simulink model "improved_hydroturbine"  (R2023b)
settings: Solver=VariableStepAuto  StartTime=0.0  StopTime=10.0  RelTol=1e-3
undefined symbols (not defined in the file or in its folder): ht
settings Model: Creator=tedbrekken  LastModifiedBy=tedbrekken

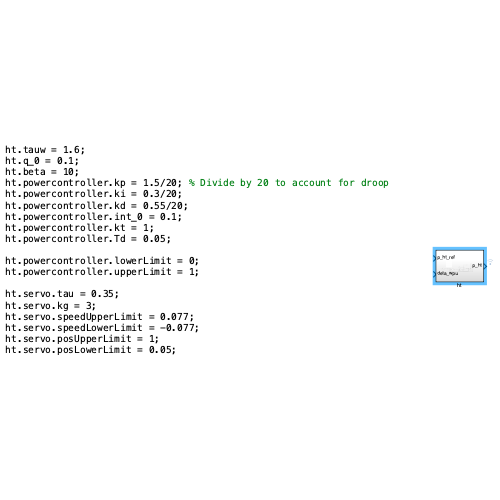
[thumbnail: Simulink's stored preview of the top-level diagram]
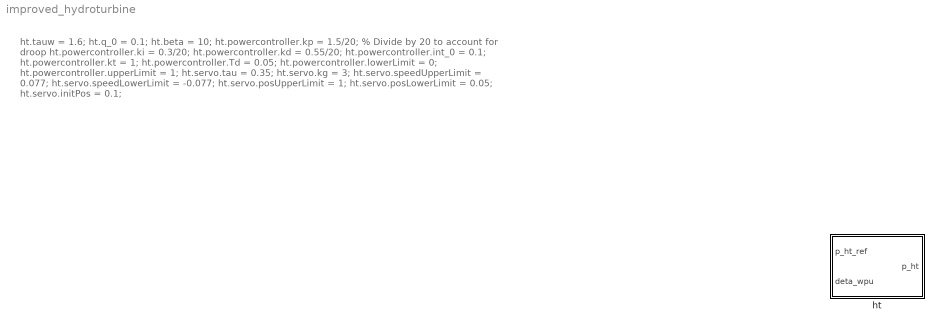
== system improved_hydroturbine ==
  note: ht.tauw = 1.6;
      | ht.q_0 = 0.1;
      | ht.beta = 10;
      | ht.powercontroller.kp = 1.5/20; % Divide by 20 to account for droop
      | ht.powercontroller.ki = 0.3/20;
      | ht.powercontroller.kd = 0.55/20;
      | ht.powercontroller.int_0 = 0.1;
      | ht.powercontroller.kt = 1;
      | ht.powercontroller.Td = 0.05;
      |
      | ht.powercontroller.lowerLimit = 0;
      | ht.powercontroller.upperLimit = 1;
      |
      | ht.servo.tau = 0.35;
      | ht.servo.kg = 3;
      | ht.servo.speedUpperLimit = 0.077;
      | ht.servo.speedLowerLimit = -0.077;
      | ht.servo.posUpperLimit = 1;
      | ht.servo.posLowerLimit = 0.05;
      | ht.servo.initPos = 0.1;
  ht : Subsystem

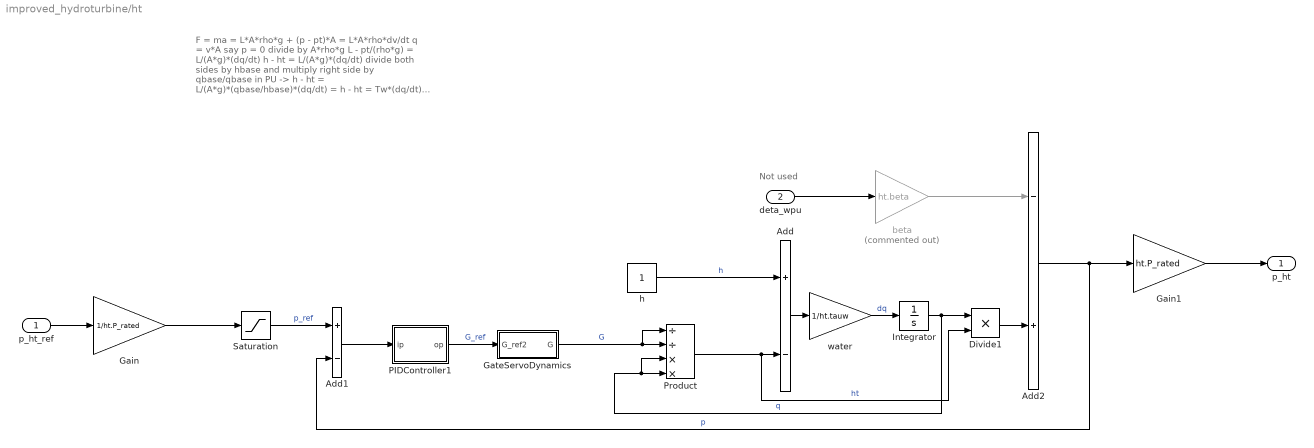
== system improved_hydroturbine/ht ==
  note: Not used
  note: F = ma = L*A*rho*g + (p - pt)*A = L*A*rho*dv/dt
      |
      | q = v*A
      |
      | say p = 0
      |
      | divide by A*rho*g
      |
      | L - pt/(rho*g) = L/(A*g)*(dq/dt)
      |
      | h - ht = L/(A*g)*(dq/dt)
      |
      | divide both sides by hbase and multiply right side by qbase/qbase
      |
      | in PU -> h - ht = L/(A*g)*(qbase/hbase)*(dq/dt) = h - ht = Tw*(dq/dt)
      |
      | ht = (q/G)^2
      |
      | pt = ht*q - beta*delta_w
      |
      | Increase in speed changes decreases relative angle of water attack on runner and decreases power
      | and vice versa
  p_ht_ref : Inport
  deta_wpu : Inport  Port=2
  Add : Sum  Inputs=+-
  Add1 : Sum  Inputs=+-
  Add2 : Sum  Inputs=-+
  Divide1 : Product  Inputs=**
  Gain : Gain  Gain=1/ht.P_rated
  Gain1 : Gain  Gain=ht.P_rated
  GateServoDynamics : Subsystem
  Integrator : Integrator  InitialCondition=ht.q_0
  PIDController1 : Subsystem  mask{kp=ht.powercontroller.kp, ki=ht.powercontroller.ki, kd=ht.powercontroller.kd, kt=ht.powercontroller.kt, Td=ht.powercontroller.Td, upperLimit=ht.powercontroller.upperLimit, lowerLimit=ht.powercontroller.lowerLimit, int_0=ht.powercontroller.int_0}
      mask prompts: kp "Proportional gain"; ki "Integral gain"; kd "Derivative gain"; kt "Windup gain"; Td "Derivative time constant"; upperLimit "Upper limit"; lowerLimit "Lower limit"; int_0 "Initial condition"
  Product : Product  Inputs=//**
  Saturation : Saturate  UpperLimit=1  LowerLimit=0
  beta : Gain  Commented=on  Gain=ht.beta
  h : Constant
  water : Gain  Gain=1/ht.tauw
  p_ht : Outport
  wires:
  water/1 -> Integrator/1  "dq"
  deta_wpu/1 -> beta/1
  beta/1 -> Add2/1
  Integrator/1 -> Product/3, Product/4, Divide1/1  "q"
  GateServoDynamics/1(G) -> Product/1, Product/2  "G"
  Product/1 -> Divide1/2, Add/2  "ht"
  Add/1 -> water/1
  h/1 -> Add/1  "h"
  Divide1/1 -> Add2/2
  PIDController1/1(op) -> GateServoDynamics/1(G_ref2)  "G_ref"
  Add2/1 -> Add1/2, Gain1/1  "p"
  Gain1/1 -> p_ht/1
  p_ht_ref/1 -> Gain/1
  Saturation/1 -> Add1/1  "p_ref"
  Gain/1 -> Saturation/1
  Add1/1 -> PIDController1/1(ip)

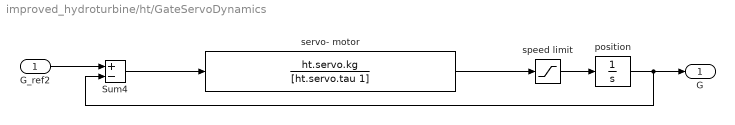
== system improved_hydroturbine/ht/GateServoDynamics ==
  G_ref2 : Inport
  Sum4 : Sum  Inputs=+-  InputSameDT=on  SaturateOnIntegerOverflow=on  OutDataTypeStr=Inherit: Same as first input
  position : Integrator  InitialCondition=ht.servo.initPos  LimitOutput=on  UpperSaturationLimit=ht.servo.posUpperLimit  LowerSaturationLimit=ht.servo.posLowerLimit
  servo- motor : TransferFcn  Numerator=ht.servo.kg  Denominator=[ht.servo.tau 1]
  speed limit : Saturate  UpperLimit=ht.servo.speedUpperLimit  LowerLimit=ht.servo.speedLowerLimit
  G : Outport
  wires:
  position/1 -> G/1, Sum4/2
  speed limit/1 -> position/1
  servo- motor/1 -> speed limit/1
  Sum4/1 -> servo- motor/1
  G_ref2/1 -> Sum4/1

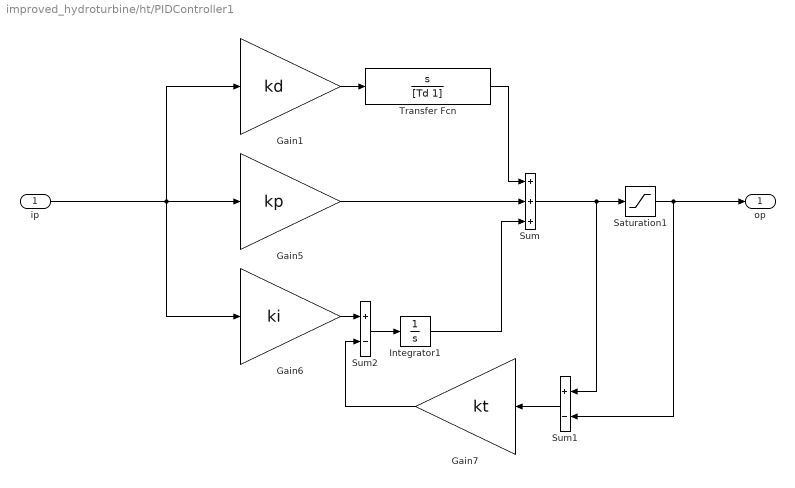
== system improved_hydroturbine/ht/PIDController1 ==
  ip : Inport
  Gain1 : Gain  Gain=kd
  Gain5 : Gain  Gain=kp
  Gain6 : Gain  Gain=ki
  Gain7 : Gain  Gain=kt
  Integrator1 : Integrator  InitialCondition=int_0
  Saturation1 : Saturate  UpperLimit=upperLimit  LowerLimit=lowerLimit
  Sum : Sum  Inputs=+++
  Sum1 : Sum  Inputs=+-
  Sum2 : Sum  Inputs=+-
  Transfer Fcn : TransferFcn  Numerator=[1 0]  Denominator=[Td 1]
  op : Outport
  wires:
  Sum2/1 -> Integrator1/1
  Integrator1/1 -> Sum/3
  Gain7/1 -> Sum2/2
  Sum1/1 -> Gain7/1
  Gain6/1 -> Sum2/1
  ip/1 -> Gain1/1, Gain6/1, Gain5/1
  Saturation1/1 -> op/1, Sum1/2
  Gain5/1 -> Sum/2
  Sum/1 -> Sum1/1, Saturation1/1
  Gain1/1 -> Transfer Fcn/1
  Transfer Fcn/1 -> Sum/1
